simulink model "sim_accelerometer"  (R2024b)
settings: Solver=ode4  StartTime=t_0  StopTime=t_f  FixedStep=dt  RelTol=1e-8
settings Model: Creator=yevge  LastModifiedBy=yevge
settings DebuggingCC: AlgebraicLoopMsg=error  CheckMatrixSingularityMsg=error

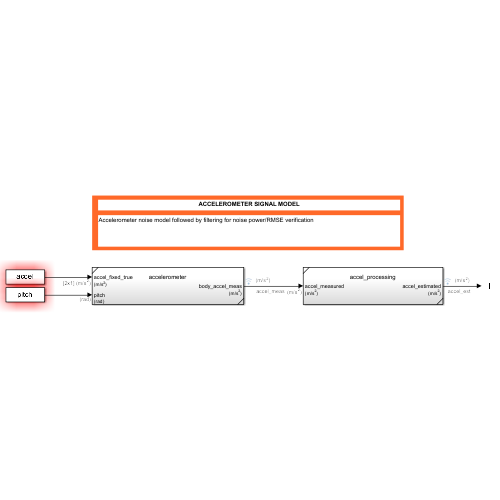
[thumbnail: Simulink's stored preview of the top-level diagram]
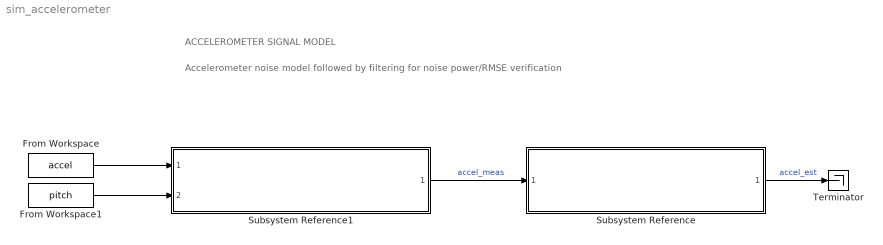
== system sim_accelerometer ==
  note: ACCELEROMETER SIGNAL MODEL
  note: Accelerometer noise model followed by filtering for noise power/RMSE verification
  From Workspace : FromWorkspace  VariableName=accel
  From Workspace1 : FromWorkspace  VariableName=pitch
  Subsystem Reference : Subsystem  ReferencedSubsystem=accel_processing
  Subsystem Reference1 : Subsystem  ReferencedSubsystem=accelerometer
  Terminator : Terminator
  wires:
  Subsystem Reference1/1 -> Subsystem Reference/1  "accel_meas"
  Subsystem Reference/1 -> Terminator/1  "accel_est"
  From Workspace/1 -> Subsystem Reference1/1
  From Workspace1/1 -> Subsystem Reference1/2
